simulink model "pi_SS_H2DF_2024a_GRU"  (R2024a)
settings: Solver=FixedStepAuto  StartTime=0.0  StopTime=inf  FixedStep=0.001  RelTol=1e-3  EnableMultiTasking=on
values from neighbouring files (symbols this model uses):
  C2C_NMPC = init_C2C_NMPC_H2DF(C2C_NMPC.expdata)    [run_SS_H2DF_control.m]
libraries: matrix_library x3, raspberrypiNetworklib x1
(part 2 of 3)

== system pi_SS_H2DF_2024a_GRU/main_C2C/Subsystem/dyn_H2DF_state_augmentation ==
  last_outputs_MC : Inport
  controls : Inport  Port=2
  last_LSTM_states : Inport  Port=3
  dyn_H2DF_state_augmentation : MATLAB Function  TreatAsAtomicUnit=on
  LSTM_states : Outport
  wires:
  dyn_H2DF_state_augmentation/1(LSTM_states) -> LSTM_states/1
  last_outputs_MC/1 -> dyn_H2DF_state_augmentation/3(last_outputs_MC)
  last_LSTM_states/1 -> dyn_H2DF_state_augmentation/1(last_LSTM_states)
  controls/1 -> dyn_H2DF_state_augmentation/2(controls)

== system pi_SS_H2DF_2024a_GRU/main_C2C/post_processing/ denormalizing reference ==
  IMEP_norm : Inport
  NOX_norm : Inport  Port=2
  soot_norm : Inport  Port=3
  MPRR_norm : Inport  Port=4
  Constant : Constant  Value=C2C_NMPC.Normalization.outputs.mean(1)
  Constant1 : Constant  Value=C2C_NMPC.Normalization.outputs.mean(2)
  Constant2 : Constant  Value=C2C_NMPC.Normalization.outputs.mean(3)
  Constant3 : Constant  Value=C2C_NMPC.Normalization.outputs.mean(4)
  Gain : Gain  Gain=C2C_NMPC.Normalization.outputs.std(1)
  Gain1 : Gain  Gain=C2C_NMPC.Normalization.outputs.std(2)
  Gain2 : Gain  Gain=C2C_NMPC.Normalization.outputs.std(3)
  Gain3 : Gain  Gain=C2C_NMPC.Normalization.outputs.std(4)
  Sum{1..3,5} (4 alike) : Sum  Inputs=|++
  IMEP : Outport
  NOX : Outport  Port=2
  soot : Outport  Port=3
  MPRR : Outport  Port=4
  wires:
  Gain/1 -> Sum5/1
  IMEP_norm/1 -> Gain/1
  Constant/1 -> Sum5/2
  Sum5/1 -> IMEP/1
  Gain1/1 -> Sum1/1
  Constant1/1 -> Sum1/2
  NOX_norm/1 -> Gain1/1
  Sum1/1 -> NOX/1
  Gain2/1 -> Sum2/1
  Constant2/1 -> Sum2/2
  soot_norm/1 -> Gain2/1
  Sum2/1 -> soot/1
  Gain3/1 -> Sum3/1
  Constant3/1 -> Sum3/2
  MPRR_norm/1 -> Gain3/1
  Sum3/1 -> MPRR/1

== system pi_SS_H2DF_2024a_GRU/main_C2C/post_processing/Subsystem1 ==
  controller_ status : Inport
  Last_Output_MC : Inport  Port=2
  " denormalizing reference" : Subsystem
  Demux : Demux
  Mux : Mux
  Mux1 : Mux  Inputs=2
  Mux2 : Mux
  Selector1 : Selector  IndexOptions=Index vector (dialog)  Indices=[(4 + C2C_NMPC.Dims.n_controls * C2C_NMPC.Opts.N + 1 * (C2C_NMPC.Dims.n_states) + C2C_NMPC.Dims.n_LSTM_states + C2C_NMPC.Dims.n_controls +1):( 4 + C2C_NMPC.Dims.n_controls * C2C_NMPC.Opts.N + 2* C2C_NMPC.Dims.n_states)]  OutputSizes=1
  Selector2 : Selector  IndexOptions=Index vector (dialog)  Indices=[(4 + C2C_NMPC.Dims.n_controls * C2C_NMPC.Opts.N + 2 * (C2C_NMPC.Dims.n_states) + C2C_NMPC.Dims.n_LSTM_states + C2C_NMPC.Dims.n_controls +1):( 4 + C2C_NMPC.Dims.n_controls * C2C_NMPC.Opts.N + 3* C2C_NMPC.Dims.n_states)]  OutputSizes=1
  Selector3 : Selector  IndexOptions=Index vector (dialog)  Indices=[(4 + C2C_NMPC.Dims.n_controls * C2C_NMPC.Opts.N + 1* (C2C_NMPC.Dims.n_LSTM_states + C2C_NMPC.Dims.n_controls) +1) : (4 + C2C_NMPC.Dims.n_controls * C2C_NMPC.Opts.N + 1* C2C_NMPC.Dims.n_states)]  OutputSizes=1
  Selector4 : Selector  IndexOptions=Index vector (dialog)  Indices=[(4 + C2C_NMPC.Dims.n_controls * C2C_NMPC.Opts.N + 3 * (C2C_NMPC.Dims.n_states) + C2C_NMPC.Dims.n_LSTM_states + C2C_NMPC.Dims.n_controls +1):( 4 + C2C_NMPC.Dims.n_controls * C2C_NMPC.Opts.N + 4* C2C_NMPC.Dims.n_states)]  OutputSizes=1
  Subsystem : Subsystem
  Out1 : Outport
  wires:
  Last_Output_MC/1 -> Demux/1
  controller_ status/1 -> Selector4/1, Selector2/1, Selector1/1, Selector3/1
  Mux1/1 -> Out1/1
  Mux/1 -> Mux1/2
  Demux/1 -> " denormalizing reference"/1(IMEP_norm)
  Demux/2 -> " denormalizing reference"/2(NOX_norm)
  Demux/3 -> " denormalizing reference"/3(soot_norm)
  Demux/4 -> " denormalizing reference"/4(MPRR_norm)
  " denormalizing reference"/2(NOX) -> Mux2/2
  " denormalizing reference"/1(IMEP) -> Mux2/1
  " denormalizing reference"/3(soot) -> Mux2/3
  " denormalizing reference"/4(MPRR) -> Mux2/4
  Mux2/1 -> Mux1/1
  Subsystem/1(Node_0) -> Mux/1
  Selector3/1 -> Subsystem/1(In1)
  Selector1/1 -> Subsystem/2(In2)
  Subsystem/2(Node_1) -> Mux/2
  Subsystem/3(Node_2) -> Mux/3
  Subsystem/4(Node_3) -> Mux/4
  Selector4/1 -> Subsystem/4(In4)
  Selector2/1 -> Subsystem/3(In3)

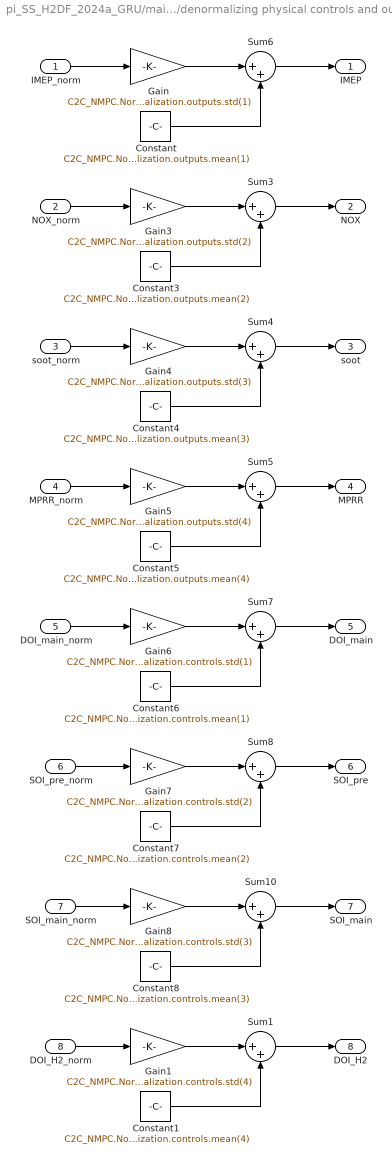
== system pi_SS_H2DF_2024a_GRU/main_C2C/post_processing/denormalizing physical controls and outputs ==
  IMEP_norm : Inport
  NOX_norm : Inport  Port=2
  soot_norm : Inport  Port=3
  MPRR_norm : Inport  Port=4
  DOI_main_norm : Inport  Port=5
  SOI_pre_norm : Inport  Port=6
  SOI_main_norm : Inport  Port=7
  DOI_H2_norm : Inport  Port=8
  Constant : Constant  Value=C2C_NMPC.Normalization.outputs.mean(1)
  Constant1 : Constant  Value=C2C_NMPC.Normalization.controls.mean(4)
  Constant3 : Constant  Value=C2C_NMPC.Normalization.outputs.mean(2)
  Constant4 : Constant  Value=C2C_NMPC.Normalization.outputs.mean(3)
  Constant5 : Constant  Value=C2C_NMPC.Normalization.outputs.mean(4)
  Constant6 : Constant  Value=C2C_NMPC.Normalization.controls.mean(1)
  Constant7 : Constant  Value=C2C_NMPC.Normalization.controls.mean(2)
  Constant8 : Constant  Value=C2C_NMPC.Normalization.controls.mean(3)
  Gain : Gain  Gain=C2C_NMPC.Normalization.outputs.std(1)
  Gain1 : Gain  Gain=C2C_NMPC.Normalization.controls.std(4)
  Gain3 : Gain  Gain=C2C_NMPC.Normalization.outputs.std(2)
  Gain4 : Gain  Gain=C2C_NMPC.Normalization.outputs.std(3)
  Gain5 : Gain  Gain=C2C_NMPC.Normalization.outputs.std(4)
  Gain6 : Gain  Gain=C2C_NMPC.Normalization.controls.std(1)
  Gain7 : Gain  Gain=C2C_NMPC.Normalization.controls.std(2)
  Gain8 : Gain  Gain=C2C_NMPC.Normalization.controls.std(3)
  Sum{1,3..8,10} (8 alike) : Sum  Inputs=|++
  IMEP : Outport
  NOX : Outport  Port=2
  soot : Outport  Port=3
  MPRR : Outport  Port=4
  DOI_main : Outport  Port=5
  SOI_pre : Outport  Port=6
  SOI_main : Outport  Port=7
  DOI_H2 : Outport  Port=8
  wires:
  Gain4/1 -> Sum4/1
  Constant3/1 -> Sum3/2
  Constant4/1 -> Sum4/2
  Gain3/1 -> Sum3/1
  Constant5/1 -> Sum5/2
  Gain5/1 -> Sum5/1
  Constant/1 -> Sum6/2
  Sum3/1 -> NOX/1
  NOX_norm/1 -> Gain3/1
  Sum5/1 -> MPRR/1
  Gain/1 -> Sum6/1
  IMEP_norm/1 -> Gain/1
  Sum6/1 -> IMEP/1
  MPRR_norm/1 -> Gain5/1
  Sum4/1 -> soot/1
  soot_norm/1 -> Gain4/1
  Constant7/1 -> Sum8/2
  Gain8/1 -> Sum10/1
  Constant6/1 -> Sum7/2
  Gain7/1 -> Sum8/1
  Sum10/1 -> SOI_main/1
  DOI_main_norm/1 -> Gain6/1
  Sum7/1 -> DOI_main/1
  Gain6/1 -> Sum7/1
  Sum8/1 -> SOI_pre/1
  Constant8/1 -> Sum10/2
  SOI_main_norm/1 -> Gain8/1
  SOI_pre_norm/1 -> Gain7/1
  Sum1/1 -> DOI_H2/1
  Constant1/1 -> Sum1/2
  Gain1/1 -> Sum1/1
  DOI_H2_norm/1 -> Gain1/1

== system pi_SS_H2DF_2024a_GRU/main_C2C/pre_processing/normalize_last_outputs_MC ==
  data_in : Inport
  Constant : Constant  Value=C2C_NMPC.Normalization.outputs.mean(1)
  Constant1 : Constant  Value=C2C_NMPC.Normalization.outputs.mean(2)
  Constant2 : Constant  Value=C2C_NMPC.Normalization.outputs.mean(3)
  Constant3 : Constant  Value=C2C_NMPC.Normalization.outputs.mean(4)
  Demux : Demux
  Gain : Gain  Gain=1/C2C_NMPC.Normalization.outputs.std(1)
  Gain1 : Gain  Gain=1/C2C_NMPC.Normalization.outputs.std(2)
  Gain2 : Gain  Gain=1/C2C_NMPC.Normalization.outputs.std(3)
  Gain3 : Gain  Gain=1/C2C_NMPC.Normalization.outputs.std(4)
  Mux : Mux
  Selector1 : Selector  IndexOptions=Index vector (dialog)  Indices=[1:4]  OutputSizes=1
  Sum{1..3,5} (4 alike) : Sum  Inputs=|+-
  last_outputs_MC : Outport  VectorParamsAs1DForOutWhenUnconnected=off
  wires:
  Demux/2 -> Sum1/1
  Constant2/1 -> Sum2/2
  Sum2/1 -> Gain2/1
  Sum1/1 -> Gain1/1
  Gain3/1 -> Mux/4
  Gain1/1 -> Mux/2
  Constant1/1 -> Sum1/2
  Demux/3 -> Sum2/1
  Gain2/1 -> Mux/3
  Mux/1 -> last_outputs_MC/1
  Constant3/1 -> Sum3/2
  Sum3/1 -> Gain3/1
  Gain/1 -> Mux/1
  Sum5/1 -> Gain/1
  Constant/1 -> Sum5/2
  Demux/1 -> Sum5/1
  data_in/1 -> Selector1/1
  Demux/4 -> Sum3/1
  Selector1/1 -> Demux/1

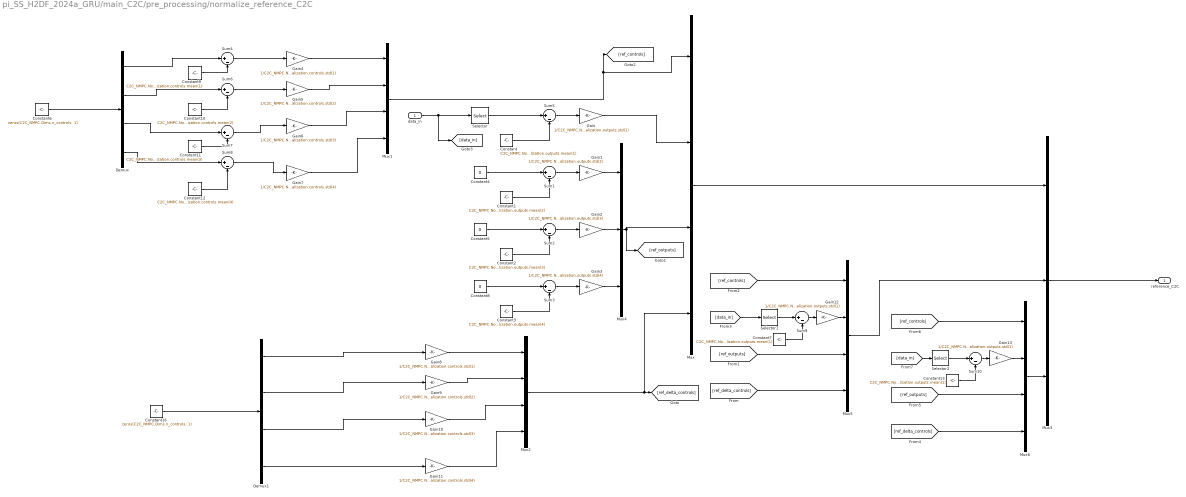
== system pi_SS_H2DF_2024a_GRU/main_C2C/pre_processing/normalize_reference_C2C ==
  data_in : Inport
  Constant : Constant  Value=C2C_NMPC.Normalization.outputs.mean(1)
  Constant1 : Constant  Value=C2C_NMPC.Normalization.outputs.mean(2)
  Constant10 : Constant  Value=C2C_NMPC.Normalization.controls.mean(2)
  Constant11 : Constant  Value=C2C_NMPC.Normalization.controls.mean(3)
  Constant12 : Constant  Value=C2C_NMPC.Normalization.controls.mean(4)
  Constant13 : Constant  Value=C2C_NMPC.Normalization.outputs.mean(1)
  Constant16 : Constant  Value=zeros(C2C_NMPC.Dims.n_controls, 1)
  Constant2 : Constant  Value=C2C_NMPC.Normalization.outputs.mean(3)
  Constant3 : Constant  Value=C2C_NMPC.Normalization.outputs.mean(4)
  Constant4 : Constant  Value=0
  Constant5 : Constant  Value=0
  Constant6 : Constant  Value=zeros(C2C_NMPC.Dims.n_controls, 1)
  Constant7 : Constant  Value=C2C_NMPC.Normalization.outputs.mean(1)
  Constant8 : Constant  Value=0
  Constant9 : Constant  Value=C2C_NMPC.Normalization.controls.mean(1)
  Demux : Demux
  Demux1 : Demux
  Gain : Gain  Gain=1/C2C_NMPC.Normalization.outputs.std(1)
  Gain1 : Gain  Gain=1/C2C_NMPC.Normalization.outputs.std(2)
  Gain10 : Gain  Gain=1/C2C_NMPC.Normalization.controls.std(3)
  Gain11 : Gain  Gain=1/C2C_NMPC.Normalization.controls.std(4)
  Gain12 : Gain  Gain=1/C2C_NMPC.Normalization.outputs.std(1)
  Gain13 : Gain  Gain=1/C2C_NMPC.Normalization.outputs.std(1)
  Gain2 : Gain  Gain=1/C2C_NMPC.Normalization.outputs.std(3)
  Gain3 : Gain  Gain=1/C2C_NMPC.Normalization.outputs.std(4)
  Gain4 : Gain  Gain=1/C2C_NMPC.Normalization.controls.std(1)
  Gain5 : Gain  Gain=1/C2C_NMPC.Normalization.controls.std(2)
  Gain6 : Gain  Gain=1/C2C_NMPC.Normalization.controls.std(3)
  Gain7 : Gain  Gain=1/C2C_NMPC.Normalization.controls.std(4)
  Gain8 : Gain  Gain=1/C2C_NMPC.Normalization.controls.std(1)
  Gain9 : Gain  Gain=1/C2C_NMPC.Normalization.controls.std(2)
  Mux{,1..2,5..6} (5 alike) : Mux
  Mux3 : Mux  Inputs=3
  Mux4 : Mux  Inputs=3
  Selector : Selector  IndexOptions=Index vector (dialog)  Indices=[5]  OutputSizes=1
  Selector1 : Selector  IndexOptions=Index vector (dialog)  Indices=7  OutputSizes=1
  Selector2 : Selector  IndexOptions=Index vector (dialog)  Indices=8  OutputSizes=1
  Sum{1..10} (10 alike) : Sum  Inputs=|+-
  reference_C2C : Outport  VectorParamsAs1DForOutWhenUnconnected=off
  wires:
  Constant/1 -> Sum5/2
  data_in/1 -> [data_in], Selector/1
  Sum5/1 -> Gain/1
  Selector/1 -> Sum5/1
  Constant4/1 -> Sum1/1
  Sum1/1 -> Gain1/1
  Constant1/1 -> Sum1/2
  Constant5/1 -> Sum2/1
  Sum2/1 -> Gain2/1
  Constant2/1 -> Sum2/2
  Constant8/1 -> Sum3/1
  Sum3/1 -> Gain3/1
  Constant3/1 -> Sum3/2
  Demux/1 -> Sum4/1
  Sum4/1 -> Gain4/1
  Constant9/1 -> Sum4/2
  Constant6/1 -> Demux/1
  Demux/2 -> Sum6/1
  Constant10/1 -> Sum6/2
  Sum6/1 -> Gain5/1
  Gain5/1 -> Mux1/2
  Gain4/1 -> Mux1/1
  Sum7/1 -> Gain6/1
  Constant11/1 -> Sum7/2
  Demux/3 -> Sum7/1
  Constant12/1 -> Sum8/2
  Sum8/1 -> Gain7/1
  Demux/4 -> Sum8/1
  Gain7/1 -> Mux1/4
  Gain6/1 -> Mux1/3
  Gain9/1 -> Mux2/2
  Gain11/1 -> Mux2/4
  Constant16/1 -> Demux1/1
  Gain8/1 -> Mux2/1
  Gain10/1 -> Mux2/3
  Demux1/4 -> Gain11/1
  Demux1/3 -> Gain10/1
  Demux1/2 -> Gain9/1
  Demux1/1 -> Gain8/1
  Mux2/1 -> [ref_delta_controls], Mux/4
  Mux3/1 -> reference_C2C/1
  Mux/1 -> Mux3/1
  Gain1/1 -> Mux4/1
  Gain2/1 -> Mux4/2
  Gain3/1 -> Mux4/3
  Gain/1 -> Mux/2
  Mux4/1 -> Mux/3, [ref_outputs]
  [ref_delta_controls] -> Mux5/4
  [ref_outputs] -> Mux5/3
  Mux1/1 -> [ref_controls], Mux/1
  [ref_controls] -> Mux5/1
  [data_in] -> Selector1/1
  Mux5/1 -> Mux3/2
  [data_in] -> Selector2/1
  [ref_controls] -> Mux6/1
  [ref_outputs] -> Mux6/3
  [ref_delta_controls] -> Mux6/4
  Mux6/1 -> Mux3/3
  Selector1/1 -> Sum9/1
  Sum9/1 -> Gain12/1
  Constant7/1 -> Sum9/2
  Gain12/1 -> Mux5/2
  Constant13/1 -> Sum10/2
  Sum10/1 -> Gain13/1
  Selector2/1 -> Sum10/1
  Gain13/1 -> Mux6/2

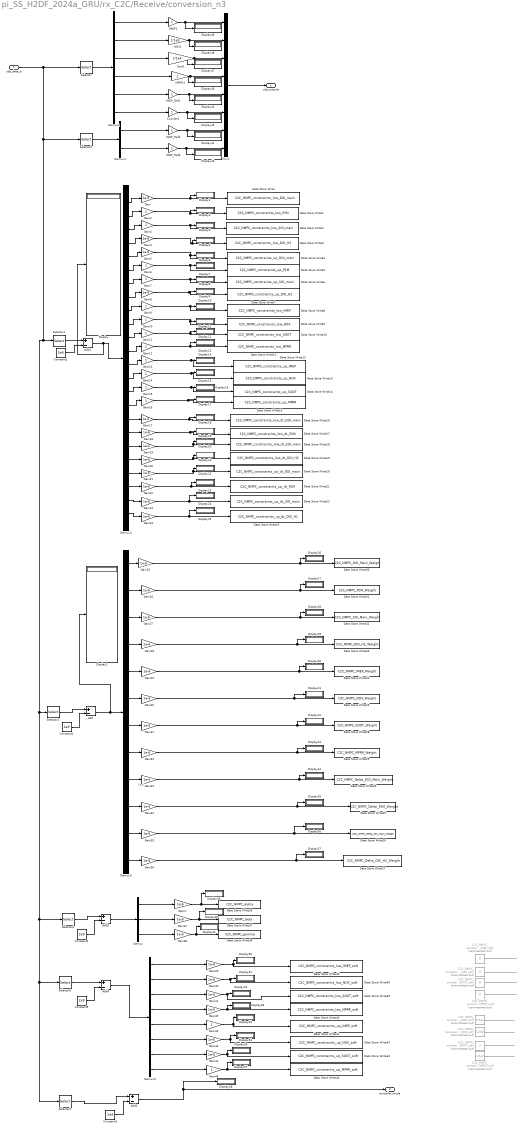
== system pi_SS_H2DF_2024a_GRU/rx_C2C/Receive/conversion_n3 ==
  note: 1e-6
  udp_data_in : Inport
  Add{,1..4} (5 alike) : Sum  Inputs=+-
  C2C_NMPC_constraints_low_IMEP_soft : Constant  Commented=on  Value=0
  C2C_NMPC_constraints_low_MPRR_soft : Constant  Commented=on  Value=0
  C2C_NMPC_constraints_low_NOX_soft : Constant  Commented=on  Value=0
  C2C_NMPC_constraints_low_SOOT_soft : Constant  Commented=on  Value=0
  C2C_NMPC_constraints_up_IMEP_soft : Constant  Commented=on  Value=9.5e5
  C2C_NMPC_constraints_up_MPRR_soft : Constant  Commented=on  Value=4.5e5
  C2C_NMPC_constraints_up_NOX_soft : Constant  Commented=on  Value=1200
  C2C_NMPC_constraints_up_SOOT_soft : Constant  Commented=on  Value=2
  Constant{1..5} (5 alike) : Constant  Value=2e9
  Counter1 : Gain
  Data Store Write : DataStoreWrite  DataStoreName=C2C_NMPC_constraints_low_DOI_main  IndexOptions=Index vector (dialog)  Indices=1  OutputSizes=1
  Data Store Write1 : DataStoreWrite  DataStoreName=C2C_NMPC_constraints_low_P2M  IndexOptions=Index vector (dialog)  Indices=1  OutputSizes=1
  Data Store Write10 : DataStoreWrite  DataStoreName=C2C_NMPC_constraints_low_SOOT  IndexOptions=Index vector (dialog)  Indices=1  OutputSizes=1
  Data Store Write11 : DataStoreWrite  DataStoreName=C2C_NMPC_constraints_low_MPRR  IndexOptions=Index vector (dialog)  Indices=1  OutputSizes=1
  Data Store Write12 : DataStoreWrite  DataStoreName=C2C_NMPC_constraints_up_IMEP  IndexOptions=Index vector (dialog)  Indices=1  OutputSizes=1
  Data Store Write13 : DataStoreWrite  DataStoreName=C2C_NMPC_constraints_up_NOX  IndexOptions=Index vector (dialog)  Indices=1  OutputSizes=1
  Data Store Write14 : DataStoreWrite  DataStoreName=C2C_NMPC_constraints_up_SOOT  IndexOptions=Index vector (dialog)  Indices=1  OutputSizes=1
  Data Store Write15 : DataStoreWrite  DataStoreName=C2C_NMPC_constraints_up_MPRR  IndexOptions=Index vector (dialog)  Indices=1  OutputSizes=1
  Data Store Write16 : DataStoreWrite  DataStoreName=C2C_NMPC_constraints_low_dt_DOI_main  IndexOptions=Index vector (dialog)  Indices=1  OutputSizes=1
  Data Store Write17 : DataStoreWrite  DataStoreName=C2C_NMPC_constraints_low_dt_P2M  IndexOptions=Index vector (dialog)  Indices=1  OutputSizes=1
  Data Store Write18 : DataStoreWrite  DataStoreName=C2C_NMPC_constraints_low_dt_SOI_main  IndexOptions=Index vector (dialog)  Indices=1  OutputSizes=1
  Data Store Write19 : DataStoreWrite  DataStoreName=C2C_NMPC_constraints_low_dt_DOI_H2  IndexOptions=Index vector (dialog)  Indices=1  OutputSizes=1
  Data Store Write2 : DataStoreWrite  DataStoreName=C2C_NMPC_constraints_low_SOI_main  IndexOptions=Index vector (dialog)  Indices=1  OutputSizes=1
  Data Store Write20 : DataStoreWrite  DataStoreName=C2C_NMPC_constraints_up_dt_DOI_main  IndexOptions=Index vector (dialog)  Indices=1  OutputSizes=1
  Data Store Write21 : DataStoreWrite  DataStoreName=C2C_NMPC_constraints_up_dt_P2M  IndexOptions=Index vector (dialog)  Indices=1  OutputSizes=1
  Data Store Write22 : DataStoreWrite  DataStoreName=C2C_NMPC_constraints_up_dt_SOI_main  IndexOptions=Index vector (dialog)  Indices=1  OutputSizes=1
  Data Store Write23 : DataStoreWrite  DataStoreName=C2C_NMPC_constraints_up_dt_DOI_H1  IndexOptions=Index vector (dialog)  Indices=1  OutputSizes=1
  Data Store Write24 : DataStoreWrite  DataStoreName=C2C_NMPC_IMEP_Weight  IndexOptions=Index vector (dialog)  Indices=1  OutputSizes=1
  Data Store Write25 : DataStoreWrite  DataStoreName=C2C_NMPC_NOX_Weight  IndexOptions=Index vector (dialog)  Indices=1  OutputSizes=1
  Data Store Write26 : DataStoreWrite  DataStoreName=C2C_NMPC_Delta_SOI_Main_Weight  IndexOptions=Index vector (dialog)  Indices=1  OutputSizes=1
  Data Store Write27 : DataStoreWrite  DataStoreName=C2C_NMPC_Delta_DOI_H2_Weight  IndexOptions=Index vector (dialog)  Indices=1  OutputSizes=1
  Data Store Write28 : DataStoreWrite  DataStoreName=C2C_NMPC_SOOT_Weight  IndexOptions=Index vector (dialog)  Indices=1  OutputSizes=1
  Data Store Write29 : DataStoreWrite  DataStoreName=C2C_NMPC_MPRR_Weight  IndexOptions=Index vector (dialog)  Indices=1  OutputSizes=1
  Data Store Write3 : DataStoreWrite  DataStoreName=C2C_NMPC_constraints_low_DOI_H2  IndexOptions=Index vector (dialog)  Indices=1  OutputSizes=1
  Data Store Write30 : DataStoreWrite  DataStoreName=C2C_NMPC_DOI_Main_Weight  IndexOptions=Index vector (dialog)  Indices=1  OutputSizes=1
  Data Store Write31 : DataStoreWrite  DataStoreName=C2C_NMPC_P2M_Weight  IndexOptions=Index vector (dialog)  Indices=1  OutputSizes=1
  Data Store Write32 : DataStoreWrite  DataStoreName=C2C_NMPC_SOI_Main_Weight  IndexOptions=Index vector (dialog)  Indices=1  OutputSizes=1
  Data Store Write33 : DataStoreWrite  DataStoreName=C2C_NMPC_DOI_H2_Weight  IndexOptions=Index vector (dialog)  Indices=1  OutputSizes=1
  Data Store Write34 : DataStoreWrite  DataStoreName=C2C_NMPC_Delta_DOI_Main_Weight  IndexOptions=Index vector (dialog)  Indices=1  OutputSizes=1
  Data Store Write35 : DataStoreWrite  DataStoreName=C2C_NMPC_Delta_P2M_Weight  IndexOptions=Index vector (dialog)  Indices=1  OutputSizes=1
  Data Store Write36 : DataStoreWrite  DataStoreName=C2C_NMPC_alpha  IndexOptions=Index vector (dialog)  Indices=1  OutputSizes=1
  Data Store Write37 : DataStoreWrite  DataStoreName=C2C_NMPC_beta  IndexOptions=Index vector (dialog)  Indices=1  OutputSizes=1
  Data Store Write38 : DataStoreWrite  DataStoreName=C2C_NMPC_gamma  IndexOptions=Index vector (dialog)  Indices=1  OutputSizes=1
  Data Store Write39 : DataStoreWrite  DataStoreName=C2C_NMPC_constraints_low_SOOT_soft  IndexOptions=Index vector (dialog)  Indices=1  OutputSizes=1
  Data Store Write4 : DataStoreWrite  DataStoreName=C2C_NMPC_constraints_up_DOI_main  IndexOptions=Index vector (dialog)  Indices=1  OutputSizes=1
  Data Store Write40 : DataStoreWrite  DataStoreName=C2C_NMPC_constraints_low_MPRR_soft  IndexOptions=Index vector (dialog)  Indices=1  OutputSizes=1
  Data Store Write41 : DataStoreWrite  DataStoreName=C2C_NMPC_constraints_up_IMEP_soft  IndexOptions=Index vector (dialog)  Indices=1  OutputSizes=1
  Data Store Write42 : DataStoreWrite  DataStoreName=C2C_NMPC_constraints_up_NOX_soft  IndexOptions=Index vector (dialog)  Indices=1  OutputSizes=1
  Data Store Write43 : DataStoreWrite  DataStoreName=C2C_NMPC_constraints_up_SOOT_soft  IndexOptions=Index vector (dialog)  Indices=1  OutputSizes=1
  Data Store Write44 : DataStoreWrite  DataStoreName=C2C_NMPC_constraints_up_MPRR_soft  IndexOptions=Index vector (dialog)  Indices=1  OutputSizes=1
  Data Store Write45 : DataStoreWrite  DataStoreName=C2C_NMPC_constraints_low_IMEP_soft  IndexOptions=Index vector (dialog)  Indices=1  OutputSizes=1
  Data Store Write46 : DataStoreWrite  DataStoreName=C2C_NMPC_constraints_low_NOX_soft  IndexOptions=Index vector (dialog)  Indices=1  OutputSizes=1
  Data Store Write5 : DataStoreWrite  DataStoreName=C2C_NMPC_constraints_up_P2M  IndexOptions=Index vector (dialog)  Indices=1  OutputSizes=1
  Data Store Write6 : DataStoreWrite  DataStoreName=C2C_NMPC_constraints_up_SOI_main  IndexOptions=Index vector (dialog)  Indices=1  OutputSizes=1
  Data Store Write7 : DataStoreWrite  DataStoreName=C2C_NMPC_constraints_up_DOI_H2  IndexOptions=Index vector (dialog)  Indices=1  OutputSizes=1
  Data Store Write8 : DataStoreWrite  DataStoreName=C2C_NMPC_constraints_low_IMEP  IndexOptions=Index vector (dialog)  Indices=1  OutputSizes=1
  Data Store Write9 : DataStoreWrite  DataStoreName=C2C_NMPC_constraints_low_NOX  IndexOptions=Index vector (dialog)  Indices=1  OutputSizes=1
  Demux : Demux  Outputs=3
  Demux1 : Demux  Outputs=6
  Demux2 : Demux  Outputs=24
  Demux3 : Demux  Outputs=12
  Demux4 : Demux  Outputs=2
  Demux5 : Demux  Outputs=8
  Display{,1..57} (58 alike) : Display
  Gain{,1,4..5,8,17..41,43..45} (33 alike) : Gain  Gain=1e-6
  Gain{2..3,6..7,9..16,42,46} (14 alike) : Gain
  IMEP1 : Gain
  IMEP_Ref1 : Gain
  IMEP_Ref2 : Gain
  IMEP_Ref3 : Gain
  MPRR1 : Gain
  Mux1 : Mux  Inputs=8
  NOX1 : Gain  Gain=1/1e3
  Selector : Selector  IndexOptions=Index vector (dialog)  Indices=[1:6]  OutputSizes=1
  Selector1 : Selector  IndexOptions=Index vector (dialog)  Indices=[7:30]  OutputSizes=1
  Selector2 : Selector  IndexOptions=Index vector (dialog)  Indices=[31:42]  OutputSizes=1
  Selector3 : Selector  IndexOptions=Index vector (dialog)  Indices=[54]  OutputSizes=1
  Selector4 : Selector  IndexOptions=Index vector (dialog)  Indices=[43:45]  OutputSizes=1
  Selector5 : Selector  IndexOptions=Index vector (dialog)  Indices=[55:56]  OutputSizes=1
  Selector6 : Selector  IndexOptions=Index vector (dialog)  Indices=[46:53]  OutputSizes=1
  Soot1 : Gain  Gain=1/1e4
  udp_outputs : Outport
  controller_mode : Outport  Port=2
  wires:
  Demux2/16 -> Gain16/1
  Demux2/1 -> Gain/1
  Demux3/9 -> Gain33/1
  Demux2/9 -> Gain9/1
  Demux2/2 -> Gain2/1
  Demux3/11 -> Gain35/1
  Demux1/1 -> IMEP1/1
  Demux2/3 -> Gain3/1
  Demux2/23 -> Gain24/1
  Demux2/18 -> Gain18/1
  Demux3/2 -> Gain26/1
  Demux1/2 -> NOX1/1
  Demux2/12 -> Gain12/1
  Demux2/19 -> Gain19/1
  Demux2/21 -> Gain21/1
  Demux1/3 -> Soot1/1
  Demux3/3 -> Gain27/1
  Demux2/15 -> Gain15/1
  Demux2/7 -> Gain7/1
  Demux3/10 -> Gain34/1
  Demux2/10 -> Gain10/1
  Demux3/8 -> Gain32/1
  Demux2/4 -> Gain4/1
  Demux2/22 -> Gain22/1
  Demux2/13 -> Gain13/1
  Demux2/14 -> Gain14/1
  Demux2/20 -> Gain20/1
  Demux2/11 -> Gain11/1
  Demux2/5 -> Gain5/1
  Selector/1 -> Demux1/1
  Demux3/6 -> Gain30/1
  Demux2/6 -> Gain6/1
  Mux1/1 -> udp_outputs/1
  Demux2/17 -> Gain17/1
  Demux2/24 -> Gain23/1
  Demux2/8 -> Gain8/1
  Demux3/4 -> Gain28/1
  Demux1/4 -> MPRR1/1
  Demux3/7 -> Gain31/1
  Demux3/1 -> Gain25/1
  Demux1/6 -> Counter1/1
  Counter1/1 -> Display45/1, Mux1/6
  NOX1/1 -> Display48/1, Mux1/2
  Soot1/1 -> Display47/1, Mux1/3
  Demux3/12 -> Gain36/1
  Demux1/5 -> IMEP_Ref1/1
  IMEP1/1 -> Display49/1, Mux1/1
  Demux3/5 -> Gain29/1
  Add/1 -> Display1/1, Demux3/1
  Constant1/1 -> Add/2
  Gain/1 -> Display2/1, Data Store Write/1
  Gain2/1 -> Display3/1, Data Store Write1/1
  Gain3/1 -> Data Store Write2/1, Display5/1
  Gain4/1 -> Display4/1, Data Store Write3/1
  Gain5/1 -> Display6/1, Data Store Write4/1
  Gain6/1 -> Display7/1, Data Store Write5/1
  Gain7/1 -> Display8/1, Data Store Write6/1
  Gain8/1 -> Display9/1, Data Store Write7/1
  Gain9/1 -> Display10/1, Data Store Write8/1
  Gain10/1 -> Display11/1, Data Store Write9/1
  Gain11/1 -> Display12/1, Data Store Write10/1
  Gain12/1 -> Display13/1, Data Store Write11/1
  Gain13/1 -> Data Store Write12/1, Display14/1
  Gain14/1 -> Display15/1, Data Store Write13/1
  Gain15/1 -> Data Store Write14/1, Display16/1
  Gain16/1 -> Display17/1, Data Store Write15/1
  Gain17/1 -> Display18/1, Data Store Write16/1
  Gain18/1 -> Display19/1, Data Store Write17/1
  Gain19/1 -> Display20/1, Data Store Write18/1
  Gain20/1 -> Display21/1, Data Store Write19/1
  Gain21/1 -> Display22/1, Data Store Write20/1
  Gain22/1 -> Display23/1, Data Store Write21/1
  Gain23/1 -> Display25/1, Data Store Write23/1
  Gain24/1 -> Display24/1, Data Store Write22/1
  Gain25/1 -> Display26/1, Data Store Write30/1
  Gain26/1 -> Display27/1, Data Store Write31/1
  Gain27/1 -> Display28/1, Data Store Write32/1
  Gain28/1 -> Display29/1, Data Store Write33/1
  Gain29/1 -> Display30/1, Data Store Write24/1
  Gain30/1 -> Display31/1, Data Store Write25/1
  Gain31/1 -> Display32/1, Data Store Write28/1
  Gain32/1 -> Display33/1, Data Store Write29/1
  Gain33/1 -> Display34/1, Data Store Write34/1
  Gain34/1 -> Display35/1, Data Store Write35/1
  Gain35/1 -> Display36/1, Data Store Write26/1
  Gain36/1 -> Display37/1, Data Store Write27/1
  Selector2/1 -> Add/1
  Selector1/1 -> Add1/1
  Add1/1 -> Display/1, Demux2/1
  Constant2/1 -> Add1/2
  Constant3/1 -> Add2/2
  Selector3/1 -> Add2/1
  Add2/1 -> controller_mode/1, Display38/1
  Constant4/1 -> Add3/2
  Selector4/1 -> Add3/1
  Add3/1 -> Demux/1
  Demux/1 -> Gain1/1
  Demux/2 -> Gain37/1
  Demux/3 -> Gain38/1
  Gain37/1 -> Display40/1, Data Store Write37/1
  Gain1/1 -> Display39/1, Data Store Write36/1
  Gain38/1 -> Display41/1, Data Store Write38/1
  IMEP_Ref2/1 -> Display42/1, Mux1/7
  IMEP_Ref3/1 -> Display43/1, Mux1/8
  Selector5/1 -> Demux4/1
  Demux4/2 -> IMEP_Ref3/1
  Demux4/1 -> IMEP_Ref2/1
  IMEP_Ref1/1 -> Mux1/5, Display44/1
  C2C_NMPC_constraints_low_SOOT_soft/1 -> ?
  C2C_NMPC_constraints_up_SOOT_soft/1 -> ?
  C2C_NMPC_constraints_up_MPRR_soft/1 -> ?
  C2C_NMPC_constraints_low_NOX_soft/1 -> ?
  C2C_NMPC_constraints_low_MPRR_soft/1 -> ?
  C2C_NMPC_constraints_up_NOX_soft/1 -> ?
  C2C_NMPC_constraints_up_IMEP_soft/1 -> ?
  C2C_NMPC_constraints_low_IMEP_soft/1 -> ?
  Gain41/1 -> Data Store Write39/1, Display52/1
  Gain39/1 -> Data Store Write45/1, Display50/1
  Gain40/1 -> Display51/1, Data Store Write46/1
  Demux5/3 -> Gain41/1
  Demux5/2 -> Gain40/1
  Demux5/1 -> Gain39/1
  Add4/1 -> Demux5/1
  Selector6/1 -> Add4/1
  Constant5/1 -> Add4/2
  udp_data_in/1 -> Selector5/1, Selector3/1, Selector6/1, Selector4/1, Selector2/1, Selector1/1, Selector/1
  Gain43/1 -> Data Store Write42/1, Display54/1
  Gain42/1 -> Display53/1, Data Store Write41/1
  Gain44/1 -> Data Store Write43/1, Display55/1
  Gain45/1 -> Display56/1, Data Store Write40/1
  Gain46/1 -> Data Store Write44/1, Display57/1
  Demux5/4 -> Gain45/1
  Demux5/5 -> Gain42/1
  Demux5/6 -> Gain43/1
  Demux5/7 -> Gain44/1
  Demux5/8 -> Gain46/1
  MPRR1/1 -> Display46/1, Mux1/4

== system pi_SS_H2DF_2024a_GRU/main_C2C/C2C_NMPC_n3/constraints no soft/Normalizing data ==
  physical_data : Inport
  Constant1 : Constant  Value=C2C_NMPC.Normalization.controls.mean(2)
  Constant2 : Constant  Value=C2C_NMPC.Normalization.controls.mean(3)
  Constant3 : Constant  Value=C2C_NMPC.Normalization.controls.mean(1)
  Constant4 : Constant  Value=C2C_NMPC.Normalization.controls.mean(4)
  Gain1 : Gain  Gain=1/C2C_NMPC.Normalization.controls.std(2)
  Gain2 : Gain  Gain=1/C2C_NMPC.Normalization.controls.std(3)
  Gain3 : Gain  Gain=1/C2C_NMPC.Normalization.controls.std(4)
  Gain4 : Gain  Gain=1/C2C_NMPC.Normalization.controls.std(1)
  Mux : Mux
  Selector : Selector  IndexOptions=Index vector (dialog)  Indices=[2]  OutputSizes=1
  Selector1 : Selector  IndexOptions=Index vector (dialog)  Indices=[1]  OutputSizes=1
  Selector2 : Selector  IndexOptions=Index vector (dialog)  Indices=[3]  OutputSizes=1
  Selector3 : Selector  IndexOptions=Index vector (dialog)  Indices=[4]  OutputSizes=1
  Sum{1..4} (4 alike) : Sum  Inputs=|+-
  normalized_data : Outport
  wires:
  physical_data/1 -> Selector2/1, Selector3/1, Selector/1, Selector1/1
  Mux/1 -> normalized_data/1
  Gain3/1 -> Mux/4
  Gain2/1 -> Mux/3
  Gain1/1 -> Mux/2
  Gain4/1 -> Mux/1
  Selector1/1 -> Sum4/1
  Selector3/1 -> Sum1/1
  Constant4/1 -> Sum1/2
  Sum1/1 -> Gain3/1
  Sum2/1 -> Gain1/1
  Constant1/1 -> Sum2/2
  Selector/1 -> Sum2/1
  Sum3/1 -> Gain2/1
  Sum4/1 -> Gain4/1
  Constant2/1 -> Sum3/2
  Selector2/1 -> Sum3/1
  Constant3/1 -> Sum4/2

== system pi_SS_H2DF_2024a_GRU/main_C2C/C2C_NMPC_n3/constraints no soft/Normalizing data1 ==
  physical_data : Inport
  Constant1 : Constant  Value=C2C_NMPC.Normalization.controls.mean(2)
  Constant2 : Constant  Value=C2C_NMPC.Normalization.controls.mean(3)
  Constant3 : Constant  Value=C2C_NMPC.Normalization.controls.mean(1)
  Constant4 : Constant  Value=C2C_NMPC.Normalization.controls.mean(4)
  Gain1 : Gain  Gain=1/C2C_NMPC.Normalization.controls.std(2)
  Gain2 : Gain  Gain=1/C2C_NMPC.Normalization.controls.std(3)
  Gain3 : Gain  Gain=1/C2C_NMPC.Normalization.controls.std(4)
  Gain4 : Gain  Gain=1/C2C_NMPC.Normalization.controls.std(1)
  Mux : Mux
  Selector : Selector  IndexOptions=Index vector (dialog)  Indices=[2]  OutputSizes=1
  Selector1 : Selector  IndexOptions=Index vector (dialog)  Indices=[1]  OutputSizes=1
  Selector2 : Selector  IndexOptions=Index vector (dialog)  Indices=[3]  OutputSizes=1
  Selector3 : Selector  IndexOptions=Index vector (dialog)  Indices=[4]  OutputSizes=1
  Sum{1..4} (4 alike) : Sum  Inputs=|+-
  normalized_data : Outport
  wires:
  physical_data/1 -> Selector2/1, Selector3/1, Selector/1, Selector1/1
  Mux/1 -> normalized_data/1
  Gain3/1 -> Mux/4
  Gain2/1 -> Mux/3
  Gain1/1 -> Mux/2
  Gain4/1 -> Mux/1
  Selector1/1 -> Sum4/1
  Selector3/1 -> Sum1/1
  Constant4/1 -> Sum1/2
  Sum1/1 -> Gain3/1
  Sum2/1 -> Gain1/1
  Constant1/1 -> Sum2/2
  Selector/1 -> Sum2/1
  Sum3/1 -> Gain2/1
  Sum4/1 -> Gain4/1
  Constant2/1 -> Sum3/2
  Selector2/1 -> Sum3/1
  Constant3/1 -> Sum4/2

== system pi_SS_H2DF_2024a_GRU/main_C2C/C2C_NMPC_n3/constraints no soft/Subsystem ==
  In : Inport
  Constant : Constant  Value=C2C_NMPC.Normalization.outputs.mean(1)
  Constant1 : Constant  Value=C2C_NMPC.Normalization.outputs.mean(2)
  Constant2 : Constant  Value=C2C_NMPC.Normalization.outputs.mean(3)
  Constant3 : Constant  Value=C2C_NMPC.Normalization.outputs.mean(4)
  Demux : Demux
  Gain : Gain  Gain=1/C2C_NMPC.Normalization.outputs.std(1)
  Gain1 : Gain  Gain=1/C2C_NMPC.Normalization.outputs.std(2)
  Gain2 : Gain  Gain=1/C2C_NMPC.Normalization.outputs.std(3)
  Gain3 : Gain  Gain=1/C2C_NMPC.Normalization.outputs.std(4)
  Mux : Mux
  Sum{1..3,5} (4 alike) : Sum  Inputs=|+-
  value : Outport
  wires:
  Mux/1 -> value/1
  In/1 -> Demux/1
  Demux/4 -> Sum3/1
  Demux/2 -> Sum1/1
  Gain1/1 -> Mux/2
  Gain3/1 -> Mux/4
  Gain2/1 -> Mux/3
  Demux/1 -> Sum5/1
  Sum5/1 -> Gain/1
  Constant3/1 -> Sum3/2
  Sum3/1 -> Gain3/1
  Gain/1 -> Mux/1
  Constant2/1 -> Sum2/2
  Sum2/1 -> Gain2/1
  Demux/3 -> Sum2/1
  Sum1/1 -> Gain1/1
  Constant1/1 -> Sum1/2
  Constant/1 -> Sum5/2

== system pi_SS_H2DF_2024a_GRU/main_C2C/C2C_NMPC_n3/constraints no soft/Subsystem1 ==
  In : Inport
  Constant : Constant  Value=C2C_NMPC.Normalization.outputs.mean(1)
  Constant1 : Constant  Value=C2C_NMPC.Normalization.outputs.mean(2)
  Constant2 : Constant  Value=C2C_NMPC.Normalization.outputs.mean(3)
  Constant3 : Constant  Value=C2C_NMPC.Normalization.outputs.mean(4)
  Demux : Demux
  Gain : Gain  Gain=1/C2C_NMPC.Normalization.outputs.std(1)
  Gain1 : Gain  Gain=1/C2C_NMPC.Normalization.outputs.std(2)
  Gain2 : Gain  Gain=1/C2C_NMPC.Normalization.outputs.std(3)
  Gain3 : Gain  Gain=1/C2C_NMPC.Normalization.outputs.std(4)
  Mux : Mux
  Sum{1..3,5} (4 alike) : Sum  Inputs=|+-
  ubh_e : Outport
  wires:
  Constant/1 -> Sum5/2
  Constant1/1 -> Sum1/2
  Sum1/1 -> Gain1/1
  Demux/3 -> Sum2/1
  Sum2/1 -> Gain2/1
  Constant2/1 -> Sum2/2
  Gain/1 -> Mux/1
  Sum3/1 -> Gain3/1
  Constant3/1 -> Sum3/2
  Sum5/1 -> Gain/1
  Demux/1 -> Sum5/1
  Gain2/1 -> Mux/3
  Gain3/1 -> Mux/4
  Gain1/1 -> Mux/2
  Demux/2 -> Sum1/1
  Demux/4 -> Sum3/1
  In/1 -> Demux/1
  Mux/1 -> ubh_e/1

== system pi_SS_H2DF_2024a_GRU/main_C2C/C2C_NMPC_n3/constraints no soft/Subsystem2 ==
  In : Inport
  Demux : Demux
  Gain : Gain  Gain=1/C2C_NMPC.Normalization.controls.std(1)
  Gain1 : Gain  Gain=1/C2C_NMPC.Normalization.controls.std(2)
  Gain2 : Gain  Gain=1/C2C_NMPC.Normalization.controls.std(3)
  Gain3 : Gain  Gain=1/C2C_NMPC.Normalization.controls.std(4)
  Mux : Mux
  Out : Outport
  wires:
  Gain3/1 -> Mux/4
  Demux/4 -> Gain3/1
  Demux/3 -> Gain2/1
  Demux/2 -> Gain1/1
  Demux/1 -> Gain/1
  Mux/1 -> Out/1
  In/1 -> Demux/1
  Gain1/1 -> Mux/2
  Gain2/1 -> Mux/3
  Gain/1 -> Mux/1

== system pi_SS_H2DF_2024a_GRU/main_C2C/C2C_NMPC_n3/constraints no soft/Subsystem3 ==
  In : Inport
  Demux : Demux
  Gain : Gain  Gain=1/C2C_NMPC.Normalization.controls.std(1)
  Gain1 : Gain  Gain=1/C2C_NMPC.Normalization.controls.std(2)
  Gain2 : Gain  Gain=1/C2C_NMPC.Normalization.controls.std(3)
  Gain3 : Gain  Gain=1/C2C_NMPC.Normalization.controls.std(4)
  Mux : Mux
  Out : Outport
  wires:
  Gain3/1 -> Mux/4
  Demux/4 -> Gain3/1
  Demux/3 -> Gain2/1
  Demux/2 -> Gain1/1
  Demux/1 -> Gain/1
  Mux/1 -> Out/1
  In/1 -> Demux/1
  Gain1/1 -> Mux/2
  Gain2/1 -> Mux/3
  Gain/1 -> Mux/1

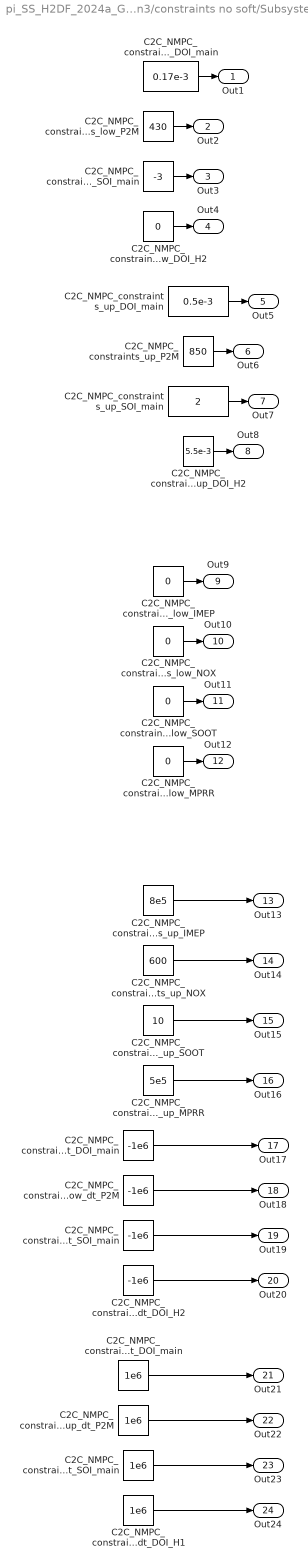
== system pi_SS_H2DF_2024a_GRU/main_C2C/C2C_NMPC_n3/constraints no soft/Subsystem4 ==
  C2C_NMPC_constraints_low_DOI_H2 : Constant  Value=0
  C2C_NMPC_constraints_low_DOI_main : Constant  Value=0.17e-3
  C2C_NMPC_constraints_low_IMEP : Constant  Value=0
  C2C_NMPC_constraints_low_MPRR : Constant  Value=0
  C2C_NMPC_constraints_low_NOX : Constant  Value=0
  C2C_NMPC_constraints_low_P2M : Constant  Value=430
  C2C_NMPC_constraints_low_SOI_main : Constant  Value=-3
  C2C_NMPC_constraints_low_SOOT : Constant  Value=0
  C2C_NMPC_constraints_low_dt_DOI_H2 : Constant  Value=-1e6
  C2C_NMPC_constraints_low_dt_DOI_main : Constant  Value=-1e6
  C2C_NMPC_constraints_low_dt_P2M : Constant  Value=-1e6
  C2C_NMPC_constraints_low_dt_SOI_main : Constant  Value=-1e6
  C2C_NMPC_constraints_up_DOI_H2 : Constant  Value=5.5e-3
  C2C_NMPC_constraints_up_DOI_main : Constant  Value=0.5e-3
  C2C_NMPC_constraints_up_IMEP : Constant  Value=8e5
  C2C_NMPC_constraints_up_MPRR : Constant  Value=5e5
  C2C_NMPC_constraints_up_NOX : Constant  Value=600
  C2C_NMPC_constraints_up_P2M : Constant  Value=850
  C2C_NMPC_constraints_up_SOI_main : Constant  Value=2
  C2C_NMPC_constraints_up_SOOT : Constant  Value=10
  C2C_NMPC_constraints_up_dt_DOI_H1 : Constant  Value=1e6
  C2C_NMPC_constraints_up_dt_DOI_main : Constant  Value=1e6
  C2C_NMPC_constraints_up_dt_P2M : Constant  Value=1e6
  C2C_NMPC_constraints_up_dt_SOI_main : Constant  Value=1e6
  Out1 : Outport
  Out2 : Outport  Port=2
  Out3 : Outport  Port=3
  Out4 : Outport  Port=4
  Out5 : Outport  Port=5
  Out6 : Outport  Port=6
  Out7 : Outport  Port=7
  Out8 : Outport  Port=8
  Out9 : Outport  Port=9
  Out10 : Outport  Port=10
  Out11 : Outport  Port=11
  Out12 : Outport  Port=12
  Out13 : Outport  Port=13
  Out14 : Outport  Port=14
  Out15 : Outport  Port=15
  Out16 : Outport  Port=16
  Out17 : Outport  Port=17
  Out18 : Outport  Port=18
  Out19 : Outport  Port=19
  Out20 : Outport  Port=20
  Out21 : Outport  Port=21
  Out22 : Outport  Port=22
  Out23 : Outport  Port=23
  Out24 : Outport  Port=24
  wires:
  C2C_NMPC_constraints_low_NOX/1 -> Out10/1
  C2C_NMPC_constraints_low_IMEP/1 -> Out9/1
  C2C_NMPC_constraints_up_DOI_main/1 -> Out5/1
  C2C_NMPC_constraints_up_SOI_main/1 -> Out7/1
  C2C_NMPC_constraints_low_MPRR/1 -> Out12/1
  C2C_NMPC_constraints_low_DOI_main/1 -> Out1/1
  C2C_NMPC_constraints_low_P2M/1 -> Out2/1
  C2C_NMPC_constraints_up_P2M/1 -> Out6/1
  C2C_NMPC_constraints_low_DOI_H2/1 -> Out4/1
  C2C_NMPC_constraints_low_SOOT/1 -> Out11/1
  C2C_NMPC_constraints_up_dt_DOI_main/1 -> Out21/1
  C2C_NMPC_constraints_low_SOI_main/1 -> Out3/1
  C2C_NMPC_constraints_up_dt_P2M/1 -> Out22/1
  C2C_NMPC_constraints_up_IMEP/1 -> Out13/1
  C2C_NMPC_constraints_up_NOX/1 -> Out14/1
  C2C_NMPC_constraints_up_MPRR/1 -> Out16/1
  C2C_NMPC_constraints_up_SOOT/1 -> Out15/1
  C2C_NMPC_constraints_low_dt_SOI_main/1 -> Out19/1
  C2C_NMPC_constraints_low_dt_DOI_main/1 -> Out17/1
  C2C_NMPC_constraints_up_DOI_H2/1 -> Out8/1
  C2C_NMPC_constraints_up_dt_DOI_H1/1 -> Out24/1
  C2C_NMPC_constraints_up_dt_SOI_main/1 -> Out23/1
  C2C_NMPC_constraints_low_dt_P2M/1 -> Out18/1
  C2C_NMPC_constraints_low_dt_DOI_H2/1 -> Out20/1

== system pi_SS_H2DF_2024a_GRU/main_C2C/C2C_NMPC_n3/constraints1 soft /Normalizing data ==
  physical_data : Inport
  Constant1 : Constant  Value=C2C_NMPC.Normalization.controls.mean(2)
  Constant2 : Constant  Value=C2C_NMPC.Normalization.controls.mean(3)
  Constant3 : Constant  Value=C2C_NMPC.Normalization.controls.mean(1)
  Constant4 : Constant  Value=C2C_NMPC.Normalization.controls.mean(4)
  Gain1 : Gain  Gain=1/C2C_NMPC.Normalization.controls.std(2)
  Gain2 : Gain  Gain=1/C2C_NMPC.Normalization.controls.std(3)
  Gain3 : Gain  Gain=1/C2C_NMPC.Normalization.controls.std(4)
  Gain4 : Gain  Gain=1/C2C_NMPC.Normalization.controls.std(1)
  Mux : Mux
  Selector : Selector  IndexOptions=Index vector (dialog)  Indices=[2]  OutputSizes=1
  Selector1 : Selector  IndexOptions=Index vector (dialog)  Indices=[1]  OutputSizes=1
  Selector2 : Selector  IndexOptions=Index vector (dialog)  Indices=[3]  OutputSizes=1
  Selector3 : Selector  IndexOptions=Index vector (dialog)  Indices=[4]  OutputSizes=1
  Sum{1..4} (4 alike) : Sum  Inputs=|+-
  normalized_data : Outport
  wires:
  Constant3/1 -> Sum4/2
  Selector2/1 -> Sum3/1
  Constant2/1 -> Sum3/2
  Sum4/1 -> Gain4/1
  Sum3/1 -> Gain2/1
  Selector/1 -> Sum2/1
  Constant1/1 -> Sum2/2
  Sum2/1 -> Gain1/1
  Sum1/1 -> Gain3/1
  Constant4/1 -> Sum1/2
  Selector3/1 -> Sum1/1
  Selector1/1 -> Sum4/1
  Gain4/1 -> Mux/1
  Gain1/1 -> Mux/2
  Gain2/1 -> Mux/3
  Gain3/1 -> Mux/4
  Mux/1 -> normalized_data/1
  physical_data/1 -> Selector1/1, Selector/1, Selector3/1, Selector2/1

== system pi_SS_H2DF_2024a_GRU/main_C2C/C2C_NMPC_n3/constraints1 soft /Normalizing data Output ==
  In : Inport
  Constant : Constant  Value=C2C_NMPC.Normalization.outputs.mean(1)
  Constant1 : Constant  Value=C2C_NMPC.Normalization.outputs.mean(2)
  Constant2 : Constant  Value=C2C_NMPC.Normalization.outputs.mean(3)
  Constant3 : Constant  Value=C2C_NMPC.Normalization.outputs.mean(4)
  Demux : Demux
  Gain : Gain  Gain=1/C2C_NMPC.Normalization.outputs.std(1)
  Gain1 : Gain  Gain=1/C2C_NMPC.Normalization.outputs.std(2)
  Gain2 : Gain  Gain=1/C2C_NMPC.Normalization.outputs.std(3)
  Gain3 : Gain  Gain=1/C2C_NMPC.Normalization.outputs.std(4)
  Mux : Mux
  Sum{1..3,5} (4 alike) : Sum  Inputs=|+-
  value : Outport
  wires:
  Constant/1 -> Sum5/2
  Constant1/1 -> Sum1/2
  Sum1/1 -> Gain1/1
  Demux/3 -> Sum2/1
  Sum2/1 -> Gain2/1
  Constant2/1 -> Sum2/2
  Gain/1 -> Mux/1
  Sum3/1 -> Gain3/1
  Constant3/1 -> Sum3/2
  Sum5/1 -> Gain/1
  Demux/1 -> Sum5/1
  Gain2/1 -> Mux/3
  Gain3/1 -> Mux/4
  Gain1/1 -> Mux/2
  Demux/2 -> Sum1/1
  Demux/4 -> Sum3/1
  In/1 -> Demux/1
  Mux/1 -> value/1

== system pi_SS_H2DF_2024a_GRU/main_C2C/C2C_NMPC_n3/constraints1 soft /Normalizing data1 ==
  physical_data : Inport
  Constant1 : Constant  Value=C2C_NMPC.Normalization.controls.mean(2)
  Constant2 : Constant  Value=C2C_NMPC.Normalization.controls.mean(3)
  Constant3 : Constant  Value=C2C_NMPC.Normalization.controls.mean(1)
  Constant4 : Constant  Value=C2C_NMPC.Normalization.controls.mean(4)
  Gain1 : Gain  Gain=1/C2C_NMPC.Normalization.controls.std(2)
  Gain2 : Gain  Gain=1/C2C_NMPC.Normalization.controls.std(3)
  Gain3 : Gain  Gain=1/C2C_NMPC.Normalization.controls.std(4)
  Gain4 : Gain  Gain=1/C2C_NMPC.Normalization.controls.std(1)
  Mux : Mux
  Selector : Selector  IndexOptions=Index vector (dialog)  Indices=[2]  OutputSizes=1
  Selector1 : Selector  IndexOptions=Index vector (dialog)  Indices=[1]  OutputSizes=1
  Selector2 : Selector  IndexOptions=Index vector (dialog)  Indices=[3]  OutputSizes=1
  Selector3 : Selector  IndexOptions=Index vector (dialog)  Indices=[4]  OutputSizes=1
  Sum{1..4} (4 alike) : Sum  Inputs=|+-
  normalized_data : Outport
  wires:
  Constant3/1 -> Sum4/2
  Selector2/1 -> Sum3/1
  Constant2/1 -> Sum3/2
  Sum4/1 -> Gain4/1
  Sum3/1 -> Gain2/1
  Selector/1 -> Sum2/1
  Constant1/1 -> Sum2/2
  Sum2/1 -> Gain1/1
  Sum1/1 -> Gain3/1
  Constant4/1 -> Sum1/2
  Selector3/1 -> Sum1/1
  Selector1/1 -> Sum4/1
  Gain4/1 -> Mux/1
  Gain1/1 -> Mux/2
  Gain2/1 -> Mux/3
  Gain3/1 -> Mux/4
  Mux/1 -> normalized_data/1
  physical_data/1 -> Selector1/1, Selector/1, Selector3/1, Selector2/1

== system pi_SS_H2DF_2024a_GRU/main_C2C/C2C_NMPC_n3/constraints1 soft /Subsystem ==
  In : Inport
  Constant : Constant  Value=C2C_NMPC.Normalization.outputs.mean(1)
  Constant1 : Constant  Value=C2C_NMPC.Normalization.outputs.mean(2)
  Constant2 : Constant  Value=C2C_NMPC.Normalization.outputs.mean(3)
  Constant3 : Constant  Value=C2C_NMPC.Normalization.outputs.mean(4)
  Demux : Demux
  Gain : Gain  Gain=1/C2C_NMPC.Normalization.outputs.std(1)
  Gain1 : Gain  Gain=1/C2C_NMPC.Normalization.outputs.std(2)
  Gain2 : Gain  Gain=1/C2C_NMPC.Normalization.outputs.std(3)
  Gain3 : Gain  Gain=1/C2C_NMPC.Normalization.outputs.std(4)
  Mux : Mux
  Sum{1..3,5} (4 alike) : Sum  Inputs=|+-
  value : Outport
  wires:
  Constant/1 -> Sum5/2
  Constant1/1 -> Sum1/2
  Sum1/1 -> Gain1/1
  Demux/3 -> Sum2/1
  Sum2/1 -> Gain2/1
  Constant2/1 -> Sum2/2
  Gain/1 -> Mux/1
  Sum3/1 -> Gain3/1
  Constant3/1 -> Sum3/2
  Sum5/1 -> Gain/1
  Demux/1 -> Sum5/1
  Gain2/1 -> Mux/3
  Gain3/1 -> Mux/4
  Gain1/1 -> Mux/2
  Demux/2 -> Sum1/1
  Demux/4 -> Sum3/1
  In/1 -> Demux/1
  Mux/1 -> value/1

== system pi_SS_H2DF_2024a_GRU/main_C2C/C2C_NMPC_n3/constraints1 soft /Subsystem1 ==
  In : Inport
  Constant : Constant  Value=C2C_NMPC.Normalization.outputs.mean(1)
  Constant1 : Constant  Value=C2C_NMPC.Normalization.outputs.mean(2)
  Constant2 : Constant  Value=C2C_NMPC.Normalization.outputs.mean(3)
  Constant3 : Constant  Value=C2C_NMPC.Normalization.outputs.mean(4)
  Demux : Demux
  Gain : Gain  Gain=1/C2C_NMPC.Normalization.outputs.std(1)
  Gain1 : Gain  Gain=1/C2C_NMPC.Normalization.outputs.std(2)
  Gain2 : Gain  Gain=1/C2C_NMPC.Normalization.outputs.std(3)
  Gain3 : Gain  Gain=1/C2C_NMPC.Normalization.outputs.std(4)
  Mux : Mux
  Sum{1..3,5} (4 alike) : Sum  Inputs=|+-
  ubh_e : Outport
  wires:
  Mux/1 -> ubh_e/1
  In/1 -> Demux/1
  Demux/4 -> Sum3/1
  Demux/2 -> Sum1/1
  Gain1/1 -> Mux/2
  Gain3/1 -> Mux/4
  Gain2/1 -> Mux/3
  Demux/1 -> Sum5/1
  Sum5/1 -> Gain/1
  Constant3/1 -> Sum3/2
  Sum3/1 -> Gain3/1
  Gain/1 -> Mux/1
  Constant2/1 -> Sum2/2
  Sum2/1 -> Gain2/1
  Demux/3 -> Sum2/1
  Sum1/1 -> Gain1/1
  Constant1/1 -> Sum1/2
  Constant/1 -> Sum5/2

== system pi_SS_H2DF_2024a_GRU/main_C2C/C2C_NMPC_n3/constraints1 soft /Subsystem2 ==
  In : Inport
  Demux : Demux
  Gain : Gain  Gain=1/C2C_NMPC.Normalization.controls.std(1)
  Gain1 : Gain  Gain=1/C2C_NMPC.Normalization.controls.std(2)
  Gain2 : Gain  Gain=1/C2C_NMPC.Normalization.controls.std(3)
  Gain3 : Gain  Gain=1/C2C_NMPC.Normalization.controls.std(4)
  Mux : Mux
  Out : Outport
  wires:
  Gain/1 -> Mux/1
  Gain2/1 -> Mux/3
  Gain1/1 -> Mux/2
  In/1 -> Demux/1
  Mux/1 -> Out/1
  Demux/1 -> Gain/1
  Demux/2 -> Gain1/1
  Demux/3 -> Gain2/1
  Demux/4 -> Gain3/1
  Gain3/1 -> Mux/4

== system pi_SS_H2DF_2024a_GRU/main_C2C/C2C_NMPC_n3/constraints1 soft /Subsystem3 ==
  In : Inport
  Demux : Demux
  Gain : Gain  Gain=1/C2C_NMPC.Normalization.controls.std(1)
  Gain1 : Gain  Gain=1/C2C_NMPC.Normalization.controls.std(2)
  Gain2 : Gain  Gain=1/C2C_NMPC.Normalization.controls.std(3)
  Gain3 : Gain  Gain=1/C2C_NMPC.Normalization.controls.std(4)
  Mux : Mux
  Out : Outport
  wires:
  Gain/1 -> Mux/1
  Gain2/1 -> Mux/3
  Gain1/1 -> Mux/2
  In/1 -> Demux/1
  Mux/1 -> Out/1
  Demux/1 -> Gain/1
  Demux/2 -> Gain1/1
  Demux/3 -> Gain2/1
  Demux/4 -> Gain3/1
  Gain3/1 -> Mux/4

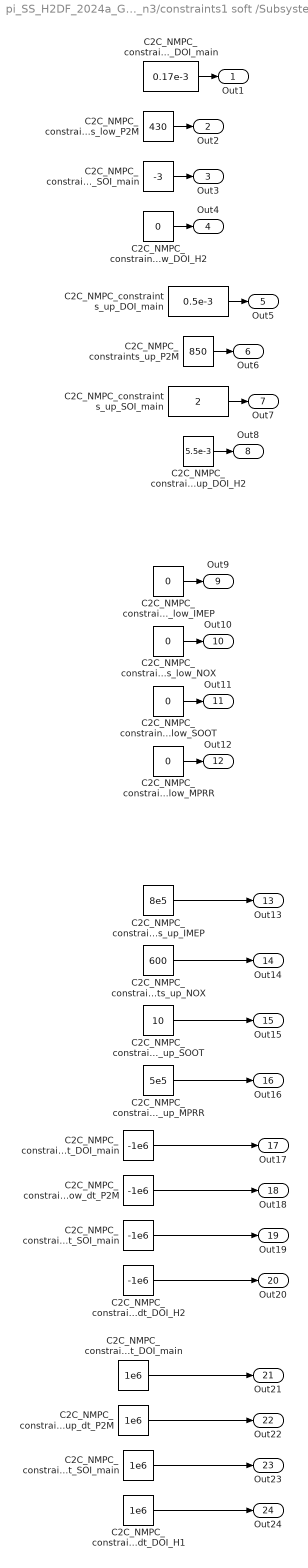
== system pi_SS_H2DF_2024a_GRU/main_C2C/C2C_NMPC_n3/constraints1 soft /Subsystem4 ==
  C2C_NMPC_constraints_low_DOI_H2 : Constant  Value=0
  C2C_NMPC_constraints_low_DOI_main : Constant  Value=0.17e-3
  C2C_NMPC_constraints_low_IMEP : Constant  Value=0
  C2C_NMPC_constraints_low_MPRR : Constant  Value=0
  C2C_NMPC_constraints_low_NOX : Constant  Value=0
  C2C_NMPC_constraints_low_P2M : Constant  Value=430
  C2C_NMPC_constraints_low_SOI_main : Constant  Value=-3
  C2C_NMPC_constraints_low_SOOT : Constant  Value=0
  C2C_NMPC_constraints_low_dt_DOI_H2 : Constant  Value=-1e6
  C2C_NMPC_constraints_low_dt_DOI_main : Constant  Value=-1e6
  C2C_NMPC_constraints_low_dt_P2M : Constant  Value=-1e6
  C2C_NMPC_constraints_low_dt_SOI_main : Constant  Value=-1e6
  C2C_NMPC_constraints_up_DOI_H2 : Constant  Value=5.5e-3
  C2C_NMPC_constraints_up_DOI_main : Constant  Value=0.5e-3
  C2C_NMPC_constraints_up_IMEP : Constant  Value=8e5
  C2C_NMPC_constraints_up_MPRR : Constant  Value=5e5
  C2C_NMPC_constraints_up_NOX : Constant  Value=600
  C2C_NMPC_constraints_up_P2M : Constant  Value=850
  C2C_NMPC_constraints_up_SOI_main : Constant  Value=2
  C2C_NMPC_constraints_up_SOOT : Constant  Value=10
  C2C_NMPC_constraints_up_dt_DOI_H1 : Constant  Value=1e6
  C2C_NMPC_constraints_up_dt_DOI_main : Constant  Value=1e6
  C2C_NMPC_constraints_up_dt_P2M : Constant  Value=1e6
  C2C_NMPC_constraints_up_dt_SOI_main : Constant  Value=1e6
  Out1 : Outport
  Out2 : Outport  Port=2
  Out3 : Outport  Port=3
  Out4 : Outport  Port=4
  Out5 : Outport  Port=5
  Out6 : Outport  Port=6
  Out7 : Outport  Port=7
  Out8 : Outport  Port=8
  Out9 : Outport  Port=9
  Out10 : Outport  Port=10
  Out11 : Outport  Port=11
  Out12 : Outport  Port=12
  Out13 : Outport  Port=13
  Out14 : Outport  Port=14
  Out15 : Outport  Port=15
  Out16 : Outport  Port=16
  Out17 : Outport  Port=17
  Out18 : Outport  Port=18
  Out19 : Outport  Port=19
  Out20 : Outport  Port=20
  Out21 : Outport  Port=21
  Out22 : Outport  Port=22
  Out23 : Outport  Port=23
  Out24 : Outport  Port=24
  wires:
  C2C_NMPC_constraints_low_dt_DOI_H2/1 -> Out20/1
  C2C_NMPC_constraints_low_dt_P2M/1 -> Out18/1
  C2C_NMPC_constraints_up_dt_SOI_main/1 -> Out23/1
  C2C_NMPC_constraints_up_dt_DOI_H1/1 -> Out24/1
  C2C_NMPC_constraints_up_DOI_H2/1 -> Out8/1
  C2C_NMPC_constraints_low_dt_DOI_main/1 -> Out17/1
  C2C_NMPC_constraints_low_dt_SOI_main/1 -> Out19/1
  C2C_NMPC_constraints_up_SOOT/1 -> Out15/1
  C2C_NMPC_constraints_up_MPRR/1 -> Out16/1
  C2C_NMPC_constraints_up_NOX/1 -> Out14/1
  C2C_NMPC_constraints_up_IMEP/1 -> Out13/1
  C2C_NMPC_constraints_up_dt_P2M/1 -> Out22/1
  C2C_NMPC_constraints_low_SOI_main/1 -> Out3/1
  C2C_NMPC_constraints_up_dt_DOI_main/1 -> Out21/1
  C2C_NMPC_constraints_low_SOOT/1 -> Out11/1
  C2C_NMPC_constraints_low_DOI_H2/1 -> Out4/1
  C2C_NMPC_constraints_up_P2M/1 -> Out6/1
  C2C_NMPC_constraints_low_P2M/1 -> Out2/1
  C2C_NMPC_constraints_low_DOI_main/1 -> Out1/1
  C2C_NMPC_constraints_low_MPRR/1 -> Out12/1
  C2C_NMPC_constraints_up_SOI_main/1 -> Out7/1
  C2C_NMPC_constraints_up_DOI_main/1 -> Out5/1
  C2C_NMPC_constraints_low_IMEP/1 -> Out9/1
  C2C_NMPC_constraints_low_NOX/1 -> Out10/1

== system pi_SS_H2DF_2024a_GRU/main_C2C/C2C_NMPC_n3/constraints1 soft /Subsystem5 ==
  In : Inport
  Constant : Constant  Value=C2C_NMPC.Normalization.outputs.mean(1)
  Constant1 : Constant  Value=C2C_NMPC.Normalization.outputs.mean(2)
  Constant2 : Constant  Value=C2C_NMPC.Normalization.outputs.mean(3)
  Constant3 : Constant  Value=C2C_NMPC.Normalization.outputs.mean(4)
  Demux : Demux
  Gain : Gain  Gain=1/C2C_NMPC.Normalization.outputs.std(1)
  Gain1 : Gain  Gain=1/C2C_NMPC.Normalization.outputs.std(2)
  Gain2 : Gain  Gain=1/C2C_NMPC.Normalization.outputs.std(3)
  Gain3 : Gain  Gain=1/C2C_NMPC.Normalization.outputs.std(4)
  Mux : Mux
  Sum{1..3,5} (4 alike) : Sum  Inputs=|+-
  ubh_e : Outport
  wires:
  Mux/1 -> ubh_e/1
  In/1 -> Demux/1
  Demux/4 -> Sum3/1
  Demux/2 -> Sum1/1
  Gain1/1 -> Mux/2
  Gain3/1 -> Mux/4
  Gain2/1 -> Mux/3
  Demux/1 -> Sum5/1
  Sum5/1 -> Gain/1
  Constant3/1 -> Sum3/2
  Sum3/1 -> Gain3/1
  Gain/1 -> Mux/1
  Constant2/1 -> Sum2/2
  Sum2/1 -> Gain2/1
  Demux/3 -> Sum2/1
  Sum1/1 -> Gain1/1
  Constant1/1 -> Sum1/2
  Constant/1 -> Sum5/2

== system pi_SS_H2DF_2024a_GRU/main_C2C/C2C_NMPC_n3/cost_function_weights/Normalize 0 to 1 ==
  In1 : Inport
  Demux : Demux
  Divide{,1..3} (4 alike) : Product  Inputs=*/
  Mux : Mux
  Sum : Sum  Inputs=|++++
  Out1 : Outport
  wires:
  Mux/1 -> Out1/1
  Divide/1 -> Mux/1
  Divide1/1 -> Mux/2
  Divide2/1 -> Mux/3
  Divide3/1 -> Mux/4
  Sum/1 -> Divide3/2, Divide2/2, Divide1/2, Divide/2
  Demux/4 -> Sum/4, Divide3/1
  Demux/3 -> Sum/3, Divide2/1
  Demux/2 -> Sum/2, Divide1/1
  Demux/1 -> Divide/1, Sum/1
  In1/1 -> Demux/1

== system pi_SS_H2DF_2024a_GRU/main_C2C/post_processing/Subsystem1/ denormalizing reference ==
  IMEP_norm : Inport
  NOX_norm : Inport  Port=2
  soot_norm : Inport  Port=3
  MPRR_norm : Inport  Port=4
  Constant : Constant  Value=C2C_NMPC.Normalization.outputs.mean(1)
  Constant1 : Constant  Value=C2C_NMPC.Normalization.outputs.mean(2)
  Constant2 : Constant  Value=C2C_NMPC.Normalization.outputs.mean(3)
  Constant3 : Constant  Value=C2C_NMPC.Normalization.outputs.mean(4)
  Gain : Gain  Gain=C2C_NMPC.Normalization.outputs.std(1)
  Gain1 : Gain  Gain=C2C_NMPC.Normalization.outputs.std(2)
  Gain2 : Gain  Gain=C2C_NMPC.Normalization.outputs.std(3)
  Gain3 : Gain  Gain=C2C_NMPC.Normalization.outputs.std(4)
  Sum{1..3,5} (4 alike) : Sum  Inputs=|++
  IMEP : Outport
  NOX : Outport  Port=2
  soot : Outport  Port=3
  MPRR : Outport  Port=4
  wires:
  Gain/1 -> Sum5/1
  IMEP_norm/1 -> Gain/1
  Constant/1 -> Sum5/2
  Sum5/1 -> IMEP/1
  Gain1/1 -> Sum1/1
  Constant1/1 -> Sum1/2
  NOX_norm/1 -> Gain1/1
  Sum1/1 -> NOX/1
  Gain2/1 -> Sum2/1
  Constant2/1 -> Sum2/2
  soot_norm/1 -> Gain2/1
  Sum2/1 -> soot/1
  Gain3/1 -> Sum3/1
  Constant3/1 -> Sum3/2
  MPRR_norm/1 -> Gain3/1
  Sum3/1 -> MPRR/1
